simulink model "ZynqBF_2tx_fpga"  (R2018b)
settings: Solver=FixedStepDiscrete  StartTime=0.0  StopTime=10.0  FixedStep=(1/420e3)/128  RelTol=1e-3
undefined symbols (not defined in the file): a, b, c, gs1_i, gs1_q, gs2_i, gs2_q, gs_length
libraries: hdlsllib x65, simulink x41
(part 4 of 4)

== matlab function ZynqBF_2tx_fpga/channel_estimator/ram_rd_counter/select_inputs ==
  data: en1 input; y output; en2 input; in1 input; in2 input
function y = fcn(en1, en2, in1, in2)
%#codegen

if (en1 && en2)
    y = zeros(1,1,'like',in1);
elseif (en1)
    y = in1;
elseif (en2)
    y = in2;
else
    y = zeros(1,1,'like',in1);
end

== matlab function ZynqBF_2tx_fpga/channel_estimator/peakdetect_ch1/correlator1/rx_ram_i/get_bit ==
  data: u input; y output; ind input
function y = fcn(u,ind)
%#codegen

y = logical(bitget(u,ind));

== matlab function ZynqBF_2tx_fpga/channel_estimator/peakdetect_ch1/correlator1/shift_rx ==
  data: u input; y output size=64; shift input [1..64]
function y = fcn(u, shift)
%#codegen
% y = zeros(64,1,'like',u);
y = circshift(u,-(int8(shift)));

== matlab function ZynqBF_2tx_fpga/channel_estimator/peakdetect_ch1/correlator1/rx_ram_q/get_bit ==
  data: u input; y output; ind input
function y = fcn(u,ind)
%#codegen

y = logical(bitget(u,ind));

== matlab function ZynqBF_2tx_fpga/channel_estimator/peakdetect_ch1/correlator1/shift_rx1 ==
  data: u input; y output size=64; shift input [1..64]
function y = fcn(u, shift)
%#codegen
% y = zeros(64,1,'like',u);
y = circshift(u,-(int8(shift)));

== matlab function ZynqBF_2tx_fpga/channel_estimator/peakdetect_ch1/correlator1/all_u ==
  data: u input size=8; y output size=1
function y = fcn(u)

y = all(u);

== matlab function ZynqBF_2tx_fpga/channel_estimator/peakdetect_ch1/correlator1/all_u1 ==
  data: u input size=8; y output size=1
function y = fcn(u)

y = all(u);

== matlab function ZynqBF_2tx_fpga/channel_estimator/ch_est/select_inputs ==
  data: en1 input; y output; en2 input; in1 input; in2 input
function y = fcn(en1, en2, in1, in2)
%#codegen

if (en1 && en2)
    y = zeros(2,1,'like',in1);
elseif (en1)
    y = in1;
elseif (en2)
    y = in2;
else
    y = zeros(2,1,'like',in1);
end

== matlab function ZynqBF_2tx_fpga/channel_estimator/peakdetect_ch2/correlator2/all_u ==
  data: u input size=8; y output size=1
function y = fcn(u)

y = all(u);

== matlab function ZynqBF_2tx_fpga/channel_estimator/peakdetect_ch2/correlator2/all_u1 ==
  data: u input size=8; y output size=1
function y = fcn(u)

y = all(u);

== matlab function ZynqBF_2tx_fpga/channel_estimator/peakdetect_ch2/correlator2/rx_ram_i/get_bit ==
  data: u input; y output; ind input
function y = fcn(u,ind)
%#codegen

y = logical(bitget(u,ind));

== matlab function ZynqBF_2tx_fpga/channel_estimator/peakdetect_ch2/correlator2/rx_ram_q/get_bit ==
  data: u input; y output; ind input
function y = fcn(u,ind)
%#codegen

y = logical(bitget(u,ind));

== matlab function ZynqBF_2tx_fpga/channel_estimator/peakdetect_ch2/correlator2/shift_rx ==
  data: u input; y output size=64; shift input [1..64]
function y = fcn(u, shift)
%#codegen
% y = zeros(64,1,'like',u);
y = circshift(u,-(int8(shift)));

== matlab function ZynqBF_2tx_fpga/channel_estimator/peakdetect_ch2/correlator2/shift_rx1 ==
  data: u input; y output size=64; shift input [1..64]
function y = fcn(u, shift)
%#codegen
% y = zeros(64,1,'like',u);
y = circshift(u,-(int8(shift)));
